simulink model "Drone_NAV_SLAM"  (R2024a)
settings: Solver=FixedStepAuto  StartTime=0.0  StopTime=inf  FixedStep=0.1  RelTol=1e-3
undefined symbols (not defined in the file or in its folder): DiscIntNeverNeededParam, gray
libraries: robotcorelib x5
settings Model: Creator=quentinlandon  LastModifiedBy=quentinlandon
settings SolverCC: AllowMultiTaskInputOutput=on  ConcurrentTasks=on
settings SFSimCC: SimTargetLang=C++

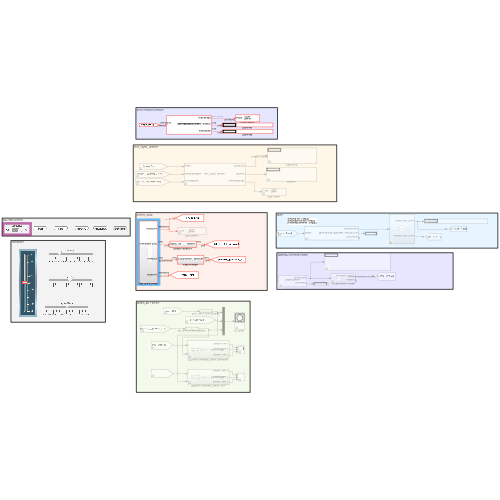
[thumbnail: Simulink's stored preview of the top-level diagram]
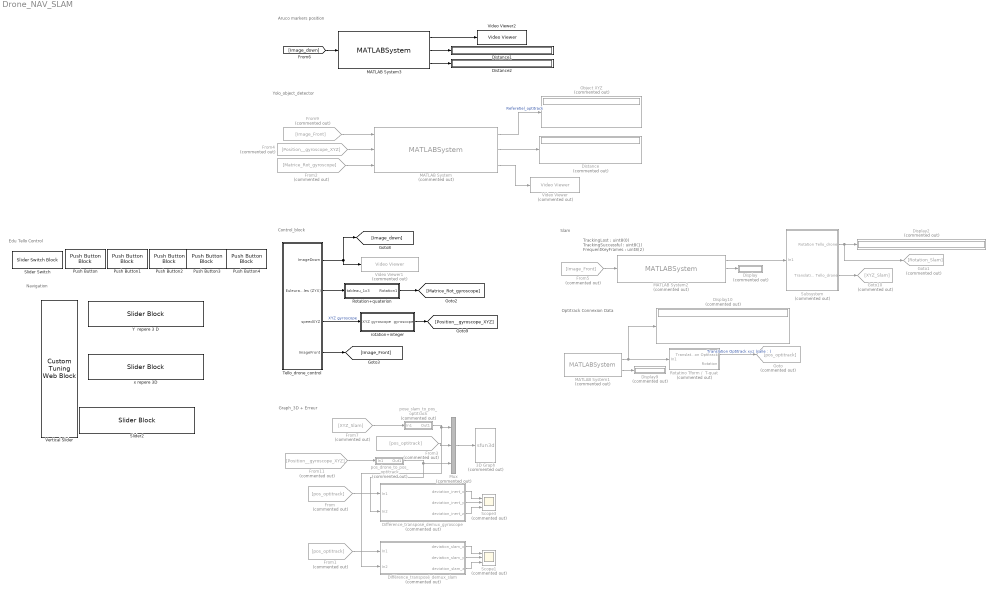
== system Drone_NAV_SLAM ==
  note: Aruco markers position
  note: Control_block
  note: Graph_3D + Erreur
  note: Slam
  note: Yolo_object_detector
  note: Optitrack Connexion Data
  note: TrackingLost : uint8(0)
      | TrackingSuccessful : uint8(1)
      | FrequentKeyFrames : uint8(2)
  note: Navigation
  note: Edu Tello Control
  3D Graph : S-Function  Commented=on  LoadFcn=if exist('sfun3d','file'), sfun3d([],[],[],'LoadBlock'); end  FunctionName=sfun3d  Parameters=ax,T,np,cp,gd,ls,mk,mx,hd,tb  SFunctionDeploymentMode=off  EnableBusSupport=off  mask(3D Graph){np=3, ax=[-5 5 -5 5 -5 5], mx=1e4, T=-1, cp=[3 2 1], gd=on, hd=off, tb=on, ls=-, mk=none}
      mask prompts: np "Number of moving points (lines)"; ax "Range: [xmin xmax  ymin ymax zmin zmax]"; mx "Max number of points in each line"; T "Sampling Time"; cp "Camera position (use [0 0 1] for 2D XY view)"; gd "Grid (on|off)"; hd "HeadMarkers (on|off)"; tb "Toolbar (on|off)"; ls "LineStyle"; mk "LineMarker"
      mask help:
      | This block plots the position of several points in the XYZ space. The input contains the coordinates of all the points (x1,y1,z1,x2,y2,z2,...).
      | The number of moving points (lines), the XYZ ranges, sampling time, camera position, and grid (among other things) can be set as mask parameters.
      settings: CopyFcn=if exist('sfun3d','file'), sfun3d([],[],[],'CopyBlock'); end  DeleteFcn=if exist('sfun3d','file'), sfun3d([],[],[],'DeleteBlock'); end  NameChangeFcn=if exist('sfun3d','file'), sfun3d([],[],[],'NameChange'); end
      mask Help:
      | This block plots the position of several points in the XYZ space. The input contains the coordinates of all the points (x1,y1,z1,x2,y2,z2,...).
      | The number of moving points (lines), the XYZ ranges, sampling time, camera position, and grid (among other things) can be set as mask parameters.
      mask TypeOptions ls: - | -- | : | -. | none
      mask TypeOptions mk: none | . | + | o | * | x | square | diamond | v | ^ | > | < | pentagram | hexagram
      mask Display: plot([.05 .95 .95 .05 .05],[.45 .45 .95 .95 .45], 0.5+cos(0:0.1:2*pi)*0.3,0.7+sin(0:0.1:2*pi)*0.2)
  Différence_transposé_demux_gyroscope : Subsystem  Commented=on
  Différence_transposé_demux_slam : Subsystem  Commented=on
  Display{,2,9..10} (4 alike) : Display  Commented=on
  Distance : Display  Commented=on
  Distance1 : Display
  Distance2 : Display
  From : From  Commented=on  GotoTag=pos_optitrack
  From1 : From  Commented=on  GotoTag=pos_optitrack
  From11 : From  Commented=on  GotoTag=Position__gyroscope_XYZ
  From2 : From  Commented=on  GotoTag=Matrice_Rot_gyroscope
  From3 : From  Commented=on  GotoTag=pos_optitrack
  From4 : From  Commented=on  GotoTag=Position__gyroscope_XYZ
  From5 : From  Commented=on  GotoTag=Image_Front
  From7 : From  Commented=on  GotoTag=XYZ_Slam
  From9 : From  Commented=on  GotoTag=Image_Front
  Goto : Goto  Commented=on  GotoTag=pos_optitrack
  Goto1 : Goto  Commented=on  GotoTag=Rotation_Slam
  Goto10 : Goto  Commented=on  GotoTag=XYZ_Slam
  MATLAB System : MATLABSystem  Commented=on  System=Yolo_Object_Detector  SimulateUsing=Interpreted execution
      mask Type: Yolo_Object_Detector
      mask Display:
      | disp('Yolo_Object_Detector');
      | port_label('input',1,'Image');
      | port_label('input',2,'TranslationMatrix');
      | port_label('input',3,'RotationMatrix');
      | port_label('output',1,'ObjectXYZ');
      | port_label('output',2,'Distance');
      | port_label('output',3,'AnnotatedImage');
  MATLAB System1 : MATLABSystem  Commented=on  System=OptilinkSystem  HostIP=10.147.125.15  ClientIP=10.147.125.15  SimulateUsing=Interpreted execution
      mask Type: OptilinkSystem
      mask Display:
      | disp('OptilinkSystem');
      | port_label('output',1,'Drones data');
      | port_label('output',2,'Connected');
  MATLAB System2 : MATLABSystem  Commented=on  System=MonoVisualSLAMSystem  FocalLength=[ 770.94, 763.00 ]  PrincipalPoint=[ 504.46, 411.48 ]  ImageSize=[ 720, 960 ]  ScaleFactor=1.2  NumLevels=6  MaxNumPoints=1500  SkipMaxFrames=10  TrackFeatureRange=[ 50, 120 ]  LoopClosureThreshold=50  Verbose=false  ThreadLevel=3  SimulateUsing=Interpreted execution
      mask Type: MonoVisualSLAMSystem
      mask Display:
      | disp('MonoVisualSLAMSystem');
      | port_label('input',1,'Image');
      | port_label('output',1,'Camera Pose');
      | port_label('output',2,'Tracking Lost');
      | port_label('output',3,'XYZ Points');
  MATLAB System3 : MATLABSystem  System=ArucoMarkerDetection  markerSizeInMM=150  markerFamily=DICT_4X4_250  maxMarkers=1  focalLength=[870,883]  principalPoint=[488,363]  imageSize=[720,960]  SimulateUsing=Interpreted execution
      mask Type: ArucoMarkerDetection
      mask Display:
      | disp('ArucoMarkerDetection');
      | port_label('input',1,'I');
      | port_label('output',1,'outputImage');
      | port_label('output',2,'cameraPositions_repere_optitrack');
      | port_label('output',3,'eulerAngles');
  Mux : Mux  Commented=on  Inputs=3
  Object XYZ : Display  Commented=on
  Push Button : PushButtonBlock  ButtonText=Takeoff  OffValue=0.000000
  Push Button1 : PushButtonBlock  ButtonText=Land  OffValue=0.000000
  Push Button2 : PushButtonBlock  ButtonText=MoveXYZ  OffValue=0.000000
  Push Button3 : PushButtonBlock  ButtonText=Moverotate  OffValue=0.000000
  Push Button4 : PushButtonBlock  ButtonText=Downcam  ButtonType=Latch  OffValue=0.000000
  Rotatino Tform /  T-quat : Subsystem  Commented=on
  Rotation+quaterion : Subsystem
  Scope1 : Scope  Commented=on  NumInputPorts=3
  Scope3 : Scope  Commented=on  NumInputPorts=3
  Slider Switch : SliderSwitchBlock
      settings: Values={{'Off', 'On'}, [0 1]}
  Slider2 : SliderBlock  ScaleMin=-180  ScaleMax=180
  Subsystem : Subsystem  Commented=on
  Tello_drone_control : Subsystem
  Vertical Slider : CustomTuningWebBlock  LabelPosition=Hide  ShowInitialText=on  Configuration="{\"components\":[{\"name\":\"LinearScaleComponent\",\"settings\":{\"bounds\":{\"max\":2,\"min\":-2,\"tickInterval\":\"auto\"},\"internalTickHeightScaleFactor\":0.5,\"labelColor\":[255,255,200],\"labelFont\":{\"font\":\"Arial\",\"fontSize\":12},\"labelOffset\":0.05,\"labelTransparency\":1,\"needleImage\":{\"size\":[596,842],\"src\":\"data:image\\/svg+xml;base64,PD94bWwgdmVyc2lvbj0iMS4wIiBlbmNvZGluZz0idXRmLTgiPz4NCjwhLS0gR2VuZXJhdG9yOiBBZG9iZSBJbGx1c3RyYXRvciAyNS4wLjAsIFNWRyBFeHBvcnQgUGx1Zy1JbiAuIFNWRyBWZXJzaW9uOiA2LjAwIEJ1aWxkIDApICAtLT4NCjxzdmcgdmVyc2lvbj0iMS4xIg0KCSBpZD0ic3ZnOCIgeG1sbnM6Y2M9Imh0dHA6Ly9jcmVhdGl2ZWNvbW1vbnMub3JnL25zIyIgeG1sbnM6ZGM9Imh0dHA6Ly9wdXJsLm9yZy9kYy9lbGVtZW50cy8xLjEvIiB4bWxuczppbmtzY2FwZT0iaHR0cDovL3d3dy5pbmtzY2FwZS5vcmcvbmFtZXNw ...(+2420 chars)\",\"srcOrientation\":\"horizontal\"},\"needleOffset\":[0.0642123287671233,-0.8044596912521441],\"needleSize\":{\"height\":0.07668067226890757,\"width\":0.4337797619047619},\"position\":[0.03623949579831933,0.2829861111111111,0.6088789682539683,0.9196428571428571],\"referencePoint\":\"auto\",\"scaleColors\":[],\"scaleColorsSize\":0.2,\"scaleDirection\":\"BT\",\"showLabels\":1,\"showMinorTicks\":0,\"showSpanLine\":1,\"showTicks\":1,\"tickColor\":[252,252,197],\"tickTransparency\":1,\"valueBarColor\":[0,114,189],\"valueBarOffset\":-0.27,\"valueBarSize\":0.1,\"valueBarTransparency\":1}},{\"name\":\"BackgroundImageComponent\",\"settings\":{\"image\":{\"size\":[380,101],\"src\":\"data:image\\/svg+xml;base64,PHN2ZyB4bWxucz0iaHR0cDovL3d3dy53My5vcmcvMjAwMC9zdmciIHhtbG5zOnhsaW5rPSJodHRwOi8vd3d3LnczLm9yZy8xOTk5L3hsaW5rIiB2aWV3Qm94PSIwIDAgMzgwIDEwMSI+PGRlZnM+PHN0eWxlPi5jbHMtMXtmaWxsOiMwMDJiNDI7fS5jbHMtMntmaWxsOiM0MjcwODI7fS5jbHMtM3tmaWxsOnVybCgjcmFkaWFsLWdyYWRpZW50KTt9LmNscy00e2ZpbGw6I2M4YzhjODtzdHJva2U6IzAwMDt9PC9zdHlsZT48cmFkaWFsR3JhZGllbnQgaWQ9InJhZGlhbC1ncmFkaWVudCIgY3g9IjE5MCIgY3k9IjUwLjUiIHI9IjI2OS4yMSIgZ3JhZGllbnRVbml0cz0idXNlclNwYWNlT25Vc2UiPjxzdG9wIG9mZnNldD0iMC4wMSIgc3RvcC1jb2xvcj0iIzNlNGY1OCIvPjxzdG9wIG9mZnNldD0iMC4wNiIgc3RvcC1jb2xvcj0iIzQ0NTc2MSIvPjxzdG9wIG9mZnNldD0iMC4xNSIgc3RvcC1jb2xvcj0iIzU1NmE3NiIvPjxzdG9wIG9mZnNldD0iMC4yNSIgc3RvcC1jb2xvcj0iIzZkODg5NSIvPjxzdG9wIG9mZnNldD0iMC4zOCIgc3RvcC1jb2xvcj0iIzhmYjJjMyIvPjxzdG9wIG9mZnNldD0iMC41MiIgc3RvcC1jb2xvcj0iI2I2ZTRmYSIvPjxzdG9wIG9mZnNldD0iMSIgc3RvcC1jb2xvcj0iIzE1NDY1NyIvPjwvcmFkaWFsR3JhZGllbnQ+PC9kZWZzPjxnIGlkPSJmcmFtZSI+PGcgaWQ9IkxheWVyXzIiIGRhdGEtbmFtZT0iTGF5ZXIgMiI+PGcgaWQ9IkxheWVyXzEtMiIgZGF0YS1uYW1lPSJMYXllciAxLTIiPjxyZWN0IGlkPSJyZWN0MTAzNiIgY2xhc3M9ImNscy0xIiB4PSIxMSIgeT0iMTEiIHdpZHRoPSIzNTgiIGhlaWdodD0iNzkiLz48cGF0aCBpZD0icGF0aDEwMzgiIGNsYXNzPSJjbHMtMiIgZD0iTTgsOFY5M0gzNzJWOFpNMzY5LDkwSDExVjExSDM2OVoiLz48cGF0aCBpZD0icGF0aDEwNDAiIGNsYXNzPSJjbHMtMyIgZD0iTTAsMFYxMDFIMzgwVjBaTTM3Miw5M0g4VjhIMzcyWiIvPjwvZz48L2c+PC9nPjxnIGlkPSJ0cmFjayI+PHBhdGggaWQ9InJlY3QxNjExIiBjbGFzcz0iY2xzLTQiIGQ9Ik0zMy4zNywyNi41OUgzNDYuNjNjNCwwLDcuMjUsMi42LDcuMjUsNS44MWgwYzAsMy4yMS0zLjI1LDUuODItNy4yNSw1LjgySDMzLjM3Yy00LDAtNy4yNS0yLjYxLTcuMjUtNS44MmgwQzI2LjEyLDI5LjE5LDI5LjM3LDI2LjU5LDMzLjM3LDI2LjU5WiIvPjwvZz48L3N2Zz4=\",\"srcOrientation\":\"horizontal\"},\"position\":[0,0,1,1],\"scaleMode\":\"0\"}},{\"name\":\"ForegroundImageComponent\",\"settings\":{\"image\":{\"size\":[0,0],\"src\":\"default\",\"srcOrientation\":[]},\"isForeground\":1,\"position\":[0,0,1,1],\"scaleMode\":\"0\"}}],\"settings\":{\"BindingType\":\"param\",\"aspectRatio\":3.7777777777777777,\"backgroundColor\":[0,0,0,\"1\"],\"backgroundOffset\":0,\"backgroundOpacity\":1,\"fixedAspectRatio\":\"on\",\"foregroundColor\":[252,252,196],\"orientation\":\"vertical\",\"showBackgroundColor\":false,\"value\":0,\"version\":\"R2023a\"},\"type\":\"LinearGauge\"}"
  Video Viewer : VideoViewer  Commented=on  colormapValue=gray(256)  FigPos=[139 735 730 455]
  Video Viewer1 : VideoViewer  Commented=on  FigPos=[-1875 839 1081 580]
  Video Viewer2 : VideoViewer  colormapValue=gray(256)  FigPos=[59 656 730 455]
  Y  repere 3 D : SliderBlock  ScaleMin=-2  ScaleMax=2
  pos_drone_to_pos_optitrack : Subsystem  Commented=on
  pose_slam_to_pos_optitrack : Subsystem  Commented=on
  rotation+integer : Subsystem
  x repere 3D : SliderBlock  ScaleMin=-2  ScaleMax=2
  wires:
  MATLAB System2/2 -> Display/1
  Subsystem/1(Rotation Tello_drone) -> Goto1/1, Display2/1
  MATLAB System1/2 -> Display9/1
  MATLAB System1/1 -> Display10/1, Rotatino Tform /  T-quat/1(In1)
  Tello_drone_control/3(speedXYZ) -> rotation+integer/1(XYZ gyroscope)  "XYZ gyroscope"
  Rotatino Tform /  T-quat/1(Translation Optitrack) -> Goto/1  "Translation Optitrack xyz (salle : )"
  Tello_drone_control/1(ImageDown) -> Video Viewer1/1, [Image_down]
  rotation+integer/1(gyroscope) -> [Position__gyroscope_XYZ]
  Subsystem/2(Translation Tello_drone) -> Goto10/1
  Mux/1 -> 3D Graph/1
  From3/1 -> Mux/2
  From/1 -> Différence_transposé_demux_gyroscope/1(In1)
  pos_drone_to_pos_optitrack/1(Out1) -> Différence_transposé_demux_gyroscope/2(In2), Mux/3
  Différence_transposé_demux_gyroscope/1(deviation_inert_x) -> Scope3/1
  Différence_transposé_demux_gyroscope/2(deviation_inert_y) -> Scope3/2
  Différence_transposé_demux_gyroscope/3(deviation_inert_z) -> Scope3/3
  From1/1 -> Différence_transposé_demux_slam/1(In1)
  pose_slam_to_pos_optitrack/1(Out1) -> Différence_transposé_demux_slam/2(In2), Mux/1
  Différence_transposé_demux_slam/1(deviation_slam_x) -> Scope1/1
  Différence_transposé_demux_slam/2(deviation_slam_y) -> Scope1/2
  Différence_transposé_demux_slam/3(deviation_slam_z) -> Scope1/3
  From5/1 -> MATLAB System2/1
  MATLAB System2/1 -> Subsystem/1(In1)
  From11/1 -> pos_drone_to_pos_optitrack/1(In1)
  From7/1 -> pose_slam_to_pos_optitrack/1(In1)
  From2/1 -> MATLAB System/3
  MATLAB System/3 -> Video Viewer/1
  From9/1 -> MATLAB System/1
  MATLAB System/2 -> Distance/1
  From4/1 -> MATLAB System/2
  Rotation+quaterion/1(Rotation1) -> [Matrice_Rot_gyroscope]
  MATLAB System/1 -> Object XYZ/1  "Referetiel_optitrack"
  [Image_down] -> MATLAB System3/1
  MATLAB System3/1 -> Video Viewer2/1
  MATLAB System3/2 -> Distance1/1
  MATLAB System3/3 -> Distance2/1
  Tello_drone_control/2(Euleurangles (ZYX)) -> Rotation+quaterion/1(tableau_1x3)
  Tello_drone_control/4(ImageFront) -> [Image_Front]

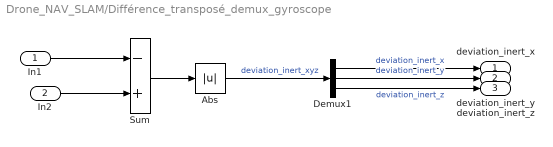
== system Drone_NAV_SLAM/Différence_transposé_demux_gyroscope ==
  In1 : Inport
  In2 : Inport  Port=2
  Abs : Abs  SaturateOnIntegerOverflow=off
  Demux1 : Demux  Outputs=3
  Sum : Sum  Inputs=-+
  deviation_inert_x : Outport
  deviation_inert_y : Outport  Port=2
  deviation_inert_z : Outport  Port=3
  wires:
  Demux1/3 -> deviation_inert_z/1  "deviation_inert_z"
  Demux1/2 -> deviation_inert_y/1  "deviation_inert_y"
  In2/1 -> Sum/2
  In1/1 -> Sum/1
  Demux1/1 -> deviation_inert_x/1  "deviation_inert_x"
  Abs/1 -> Demux1/1  "deviation_inert_xyz"
  Sum/1 -> Abs/1

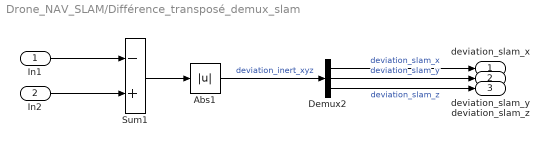
== system Drone_NAV_SLAM/Différence_transposé_demux_slam ==
  In1 : Inport
  In2 : Inport  Port=2
  Abs1 : Abs  SaturateOnIntegerOverflow=off
  Demux2 : Demux  Outputs=3
  Sum1 : Sum  Inputs=-+
  deviation_slam_x : Outport
  deviation_slam_y : Outport  Port=2
  deviation_slam_z : Outport  Port=3
  wires:
  In1/1 -> Sum1/1
  Demux2/1 -> deviation_slam_x/1  "deviation_slam_x"
  In2/1 -> Sum1/2
  Demux2/3 -> deviation_slam_z/1  "deviation_slam_z"
  Abs1/1 -> Demux2/1  "deviation_inert_xyz"
  Sum1/1 -> Abs1/1
  Demux2/2 -> deviation_slam_y/1  "deviation_slam_y"

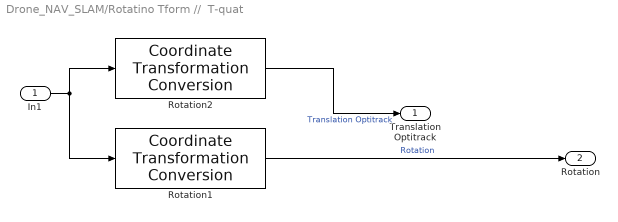
== system Drone_NAV_SLAM/Rotatino Tform //  T-quat ==
  In1 : Inport
  Rotation1 : robotcorelib/Coordinate Transformation Conversion  InputRepresentation=Homogeneous Transformation  InputEulerSequence=ZYX  ShowTrVecInputPort=on  OutputRepresentation=Quaternion  OutputEulerSequence=ZYX  ShowTrVecOutputPort=off  SimulateUsing=Code generation
      settings: LibrarySourceBlock=uavutilslib/Coordinate Transformation Conversion
  Rotation2 : robotcorelib/Coordinate Transformation Conversion  InputRepresentation=Homogeneous Transformation  InputEulerSequence=ZYX  ShowTrVecInputPort=on  OutputRepresentation=Translation Vector  OutputEulerSequence=ZYX  ShowTrVecOutputPort=off  SimulateUsing=Code generation
      settings: LibrarySourceBlock=uavutilslib/Coordinate Transformation Conversion
  Translation Optitrack : Outport
  Rotation : Outport  Port=2
  wires:
  Rotation1/1 -> Rotation/1  "Rotation"
  Rotation2/1 -> Translation Optitrack/1  "Translation Optitrack"
  In1/1 -> Rotation2/1, Rotation1/1

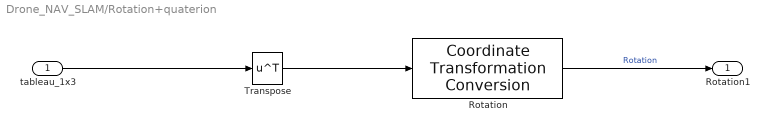
== system Drone_NAV_SLAM/Rotation+quaterion ==
  tableau_1x3 : Inport
  Rotation : robotcorelib/Coordinate Transformation Conversion  InputRepresentation=Euler Angles  InputEulerSequence=ZYX  ShowTrVecInputPort=on  OutputRepresentation=Rotation Matrix  OutputEulerSequence=ZYX  ShowTrVecOutputPort=off  SimulateUsing=Code generation
      settings: LibrarySourceBlock=uavutilslib/Coordinate Transformation Conversion
  Transpose : Math  Operator=transpose
  Rotation1 : Outport
  wires:
  Rotation/1 -> Rotation1/1  "Rotation"
  Transpose/1 -> Rotation/1
  tableau_1x3/1 -> Transpose/1

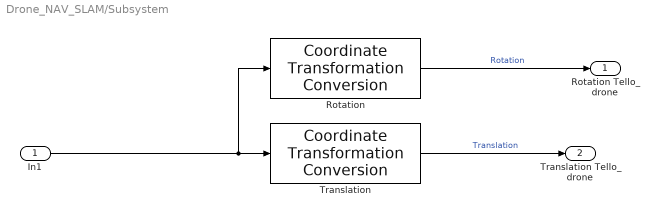
== system Drone_NAV_SLAM/Subsystem ==
  In1 : Inport
  Rotation : robotcorelib/Coordinate Transformation Conversion  InputRepresentation=Homogeneous Transformation  InputEulerSequence=ZYX  ShowTrVecInputPort=on  OutputRepresentation=Rotation Matrix  OutputEulerSequence=ZYX  ShowTrVecOutputPort=off  SimulateUsing=Code generation
      settings: LibrarySourceBlock=uavutilslib/Coordinate Transformation Conversion
  Translation : robotcorelib/Coordinate Transformation Conversion  InputRepresentation=Homogeneous Transformation  InputEulerSequence=ZYX  ShowTrVecInputPort=on  OutputRepresentation=Translation Vector  OutputEulerSequence=ZYX  ShowTrVecOutputPort=on  SimulateUsing=Code generation
      settings: LibrarySourceBlock=uavutilslib/Coordinate Transformation Conversion
  Rotation Tello_drone : Outport
  Translation Tello_drone : Outport  Port=2
  wires:
  Translation/1 -> Translation Tello_drone/1  "Translation"
  Rotation/1 -> Rotation Tello_drone/1  "Rotation"
  In1/1 -> Rotation/1, Translation/1

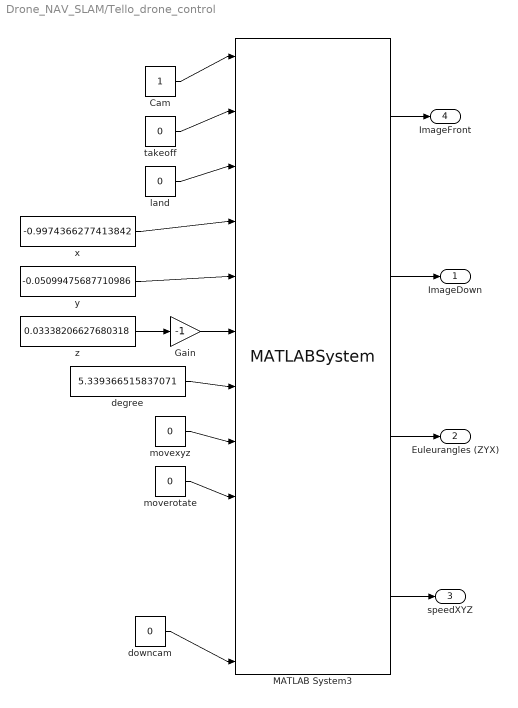
== system Drone_NAV_SLAM/Tello_drone_control ==
  Cam : Constant
  Gain : Gain  Gain=-1
  MATLAB System3 : MATLABSystem  System=Tello_drone_control  droneIP=127.0.0.1  SimulateUsing=Interpreted execution
      mask Type: Tello_drone_control
      mask Display:
      | disp('Tello_drone_control');
      | port_label('input',1,'Slam');
      | port_label('input',2,'tkoff');
      | port_label('input',3,'landing');
      | port_label('input',4,'xMove');
      | port_label('input',5,'yMove');
      | port_label('input',6,'zMove');
      | port_label('input',7,'degree');
      | port_label('input',8,'movexyz');
      | port_label('input',9,'moverotate');
      | port_label('input',10,'enableRC');
      | port_label('input',11,'rcspeeds');
      | port_label('input',12,'downcam');
      | port_label('output',1,'imageFront');
      | port_label('output',2,'imageDown');
      | port_label('output',3,'Eulerangles');
      | port_label('output',4,'speedXYZ');
  degree : Constant  Value=5.339366515837071
  downcam : Constant  Value=0
  land : Constant  Value=0
  moverotate : Constant  Value=0
  movexyz : Constant  Value=0
  takeoff : Constant  Value=0
  x : Constant  Value=-0.9974366277413842
  y : Constant  Value=-0.05099475687710986
  z : Constant  Value=0.03338206627680318
  ImageDown : Outport
  Euleurangles (ZYX) : Outport  Port=2
  speedXYZ : Outport  Port=3
  ImageFront : Outport  Port=4
  wires:
  moverotate/1 -> MATLAB System3/9
  land/1 -> MATLAB System3/3
  y/1 -> MATLAB System3/5
  x/1 -> MATLAB System3/4
  Gain/1 -> MATLAB System3/6
  z/1 -> Gain/1
  degree/1 -> MATLAB System3/7
  Cam/1 -> MATLAB System3/1
  movexyz/1 -> MATLAB System3/8
  takeoff/1 -> MATLAB System3/2
  downcam/1 -> MATLAB System3/12
  MATLAB System3/4 -> speedXYZ/1
  MATLAB System3/3 -> Euleurangles (ZYX)/1
  MATLAB System3/2 -> ImageDown/1
  MATLAB System3/1 -> ImageFront/1

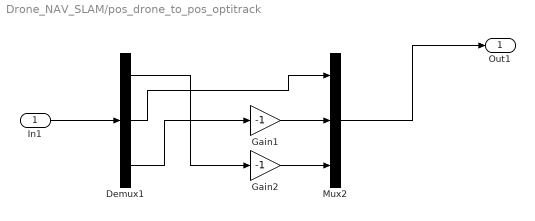
== system Drone_NAV_SLAM/pos_drone_to_pos_optitrack ==
  In1 : Inport
  Demux1 : Demux  Outputs=3
  Gain1 : Gain  Gain=-1
  Gain2 : Gain  Gain=-1
  Mux2 : Mux  Inputs=3
  Out1 : Outport
  wires:
  Demux1/1 -> Gain2/1
  In1/1 -> Demux1/1
  Mux2/1 -> Out1/1
  Gain1/1 -> Mux2/2
  Demux1/3 -> Gain1/1
  Demux1/2 -> Mux2/1
  Gain2/1 -> Mux2/3

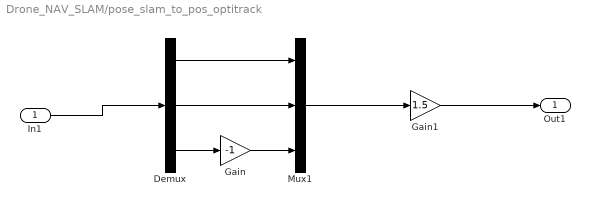
== system Drone_NAV_SLAM/pose_slam_to_pos_optitrack ==
  In1 : Inport
  Demux : Demux  Outputs=3
  Gain : Gain  Gain=-1
  Gain1 : Gain  Gain=1.5
  Mux1 : Mux  Inputs=3
  Out1 : Outport
  wires:
  Mux1/1 -> Gain1/1
  In1/1 -> Demux/1
  Demux/1 -> Mux1/1
  Demux/3 -> Gain/1
  Demux/2 -> Mux1/2
  Gain/1 -> Mux1/3
  Gain1/1 -> Out1/1

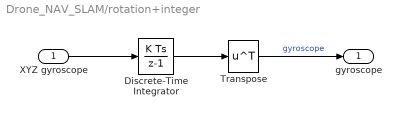
== system Drone_NAV_SLAM/rotation+integer ==
  XYZ gyroscope : Inport
  Discrete-Time Integrator : DiscreteIntegrator  SampleTime=-1  ICPrevOutput=DiscIntNeverNeededParam  ICPrevScaledInput=DiscIntNeverNeededParam
  Transpose : Math  Operator=transpose
  gyroscope : Outport
  wires:
  XYZ gyroscope/1 -> Discrete-Time Integrator/1
  Transpose/1 -> gyroscope/1  "gyroscope"
  Discrete-Time Integrator/1 -> Transpose/1
